simulink model "MCSI_simulation_2024_final_sim"  (R2021a)
settings: Solver=VariableStepAuto  StartTime=0.0  StopTime=10/cfg.fl  RelTol=1e-3
undefined symbols (not defined in the file or in its folder): cfg
libraries: spsIdealSwitchLib x18, simulink x17, hdlsllib x12, spsSeriesRLCBranchLib x8, spsCurrentMeasurementLib x6, commutil2 x6, spsMosfetLib x4, spsTriangleGeneratorLib x3, spsThreePhaseProgrammableGeneratorLib x3, spsMeanLib x2, spsThreePhaseSeriesRLCBranchLib x2, spsThreePhaseVIMeasurementLib x2
(part 2 of 2)

== system MCSI_simulation_2024_final_sim/SPWM_3mod_hdl/tabla_spwm_g1/Decoder ==
  note: LSB
  b2 : Inport
  b1 : Inport  Port=2
  b0 (LSB) : Inport  Port=3
  Logical Operator{,1..7} (8 alike) : Logic  Inputs=3  IconShape=distinctive  AllPortsSameDT=off  OutDataTypeStr=boolean
  Logical Operator10 : Logic  Operator=NOT  IconShape=distinctive  AllPortsSameDT=off  OutDataTypeStr=boolean
  Logical Operator8 : Logic  Operator=NOT  IconShape=distinctive  AllPortsSameDT=off  OutDataTypeStr=boolean
  Logical Operator9 : Logic  Operator=NOT  IconShape=distinctive  AllPortsSameDT=off  OutDataTypeStr=boolean
  Out1 : Outport
  Out2 : Outport  Port=2
  Out3 : Outport  Port=3
  Out4 : Outport  Port=4
  Out5 : Outport  Port=5
  Out6 : Outport  Port=6
  Out7 : Outport  Port=7
  Out8 : Outport  Port=8
  wires:
  Logical Operator9/1 -> Logical Operator5/2, Logical Operator4/2, Logical Operator1/2, Logical Operator/2
  Logical Operator5/1 -> Out6/1
  Logical Operator1/1 -> Out2/1
  Logical Operator10/1 -> Logical Operator3/3, Logical Operator2/3, Logical Operator/3, Logical Operator1/3
  Logical Operator/1 -> Out1/1
  Logical Operator8/1 -> Logical Operator6/1, Logical Operator4/1, Logical Operator2/1, Logical Operator/1
  b2/1 -> Logical Operator4/3, Logical Operator5/3, Logical Operator7/3, Logical Operator6/3, Logical Operator10/1
  b0 (LSB)/1 -> Logical Operator7/1, Logical Operator5/1, Logical Operator3/1, Logical Operator1/1, Logical Operator8/1
  Logical Operator7/1 -> Out8/1
  b1/1 -> Logical Operator3/2, Logical Operator2/2, Logical Operator7/2, Logical Operator6/2, Logical Operator9/1
  Logical Operator4/1 -> Out5/1
  Logical Operator6/1 -> Out7/1
  Logical Operator3/1 -> Out4/1
  Logical Operator2/1 -> Out3/1

== system MCSI_simulation_2024_final_sim/SPWM_3mod_hdl1/Maximum Calculator/Decoder ==
  note: LSB
  b2 : Inport
  b1 : Inport  Port=2
  b0 (LSB) : Inport  Port=3
  Logical Operator{,1..7} (8 alike) : Logic  Inputs=3  IconShape=distinctive  AllPortsSameDT=off  OutDataTypeStr=boolean
  Logical Operator10 : Logic  Operator=NOT  IconShape=distinctive  AllPortsSameDT=off  OutDataTypeStr=boolean
  Logical Operator8 : Logic  Operator=NOT  IconShape=distinctive  AllPortsSameDT=off  OutDataTypeStr=boolean
  Logical Operator9 : Logic  Operator=NOT  IconShape=distinctive  AllPortsSameDT=off  OutDataTypeStr=boolean
  Out1 : Outport
  Out2 : Outport  Port=2
  Out3 : Outport  Port=3
  Out4 : Outport  Port=4
  Out5 : Outport  Port=5
  Out6 : Outport  Port=6
  Out7 : Outport  Port=7
  Out8 : Outport  Port=8
  wires:
  Logical Operator9/1 -> Logical Operator5/2, Logical Operator4/2, Logical Operator1/2, Logical Operator/2
  Logical Operator5/1 -> Out6/1
  Logical Operator1/1 -> Out2/1
  Logical Operator10/1 -> Logical Operator3/3, Logical Operator2/3, Logical Operator/3, Logical Operator1/3
  Logical Operator/1 -> Out1/1
  Logical Operator8/1 -> Logical Operator6/1, Logical Operator4/1, Logical Operator2/1, Logical Operator/1
  b2/1 -> Logical Operator4/3, Logical Operator5/3, Logical Operator7/3, Logical Operator6/3, Logical Operator10/1
  b0 (LSB)/1 -> Logical Operator7/1, Logical Operator5/1, Logical Operator3/1, Logical Operator1/1, Logical Operator8/1
  Logical Operator7/1 -> Out8/1
  b1/1 -> Logical Operator3/2, Logical Operator2/2, Logical Operator7/2, Logical Operator6/2, Logical Operator9/1
  Logical Operator4/1 -> Out5/1
  Logical Operator6/1 -> Out7/1
  Logical Operator3/1 -> Out4/1
  Logical Operator2/1 -> Out3/1

== system MCSI_simulation_2024_final_sim/SPWM_3mod_hdl1/tabla_spwm_g1/Decoder ==
  note: LSB
  b2 : Inport
  b1 : Inport  Port=2
  b0 (LSB) : Inport  Port=3
  Logical Operator{,1..7} (8 alike) : Logic  Inputs=3  IconShape=distinctive  AllPortsSameDT=off  OutDataTypeStr=boolean
  Logical Operator10 : Logic  Operator=NOT  IconShape=distinctive  AllPortsSameDT=off  OutDataTypeStr=boolean
  Logical Operator8 : Logic  Operator=NOT  IconShape=distinctive  AllPortsSameDT=off  OutDataTypeStr=boolean
  Logical Operator9 : Logic  Operator=NOT  IconShape=distinctive  AllPortsSameDT=off  OutDataTypeStr=boolean
  Out1 : Outport
  Out2 : Outport  Port=2
  Out3 : Outport  Port=3
  Out4 : Outport  Port=4
  Out5 : Outport  Port=5
  Out6 : Outport  Port=6
  Out7 : Outport  Port=7
  Out8 : Outport  Port=8
  wires:
  Logical Operator9/1 -> Logical Operator5/2, Logical Operator4/2, Logical Operator1/2, Logical Operator/2
  Logical Operator5/1 -> Out6/1
  Logical Operator1/1 -> Out2/1
  Logical Operator10/1 -> Logical Operator3/3, Logical Operator2/3, Logical Operator/3, Logical Operator1/3
  Logical Operator/1 -> Out1/1
  Logical Operator8/1 -> Logical Operator6/1, Logical Operator4/1, Logical Operator2/1, Logical Operator/1
  b2/1 -> Logical Operator4/3, Logical Operator5/3, Logical Operator7/3, Logical Operator6/3, Logical Operator10/1
  b0 (LSB)/1 -> Logical Operator7/1, Logical Operator5/1, Logical Operator3/1, Logical Operator1/1, Logical Operator8/1
  Logical Operator7/1 -> Out8/1
  b1/1 -> Logical Operator3/2, Logical Operator2/2, Logical Operator7/2, Logical Operator6/2, Logical Operator9/1
  Logical Operator4/1 -> Out5/1
  Logical Operator6/1 -> Out7/1
  Logical Operator3/1 -> Out4/1
  Logical Operator2/1 -> Out3/1

== system MCSI_simulation_2024_final_sim/SPWM_3mod_hdl2/Maximum Calculator/Decoder ==
  note: LSB
  b2 : Inport
  b1 : Inport  Port=2
  b0 (LSB) : Inport  Port=3
  Logical Operator{,1..7} (8 alike) : Logic  Inputs=3  IconShape=distinctive  AllPortsSameDT=off  OutDataTypeStr=boolean
  Logical Operator10 : Logic  Operator=NOT  IconShape=distinctive  AllPortsSameDT=off  OutDataTypeStr=boolean
  Logical Operator8 : Logic  Operator=NOT  IconShape=distinctive  AllPortsSameDT=off  OutDataTypeStr=boolean
  Logical Operator9 : Logic  Operator=NOT  IconShape=distinctive  AllPortsSameDT=off  OutDataTypeStr=boolean
  Out1 : Outport
  Out2 : Outport  Port=2
  Out3 : Outport  Port=3
  Out4 : Outport  Port=4
  Out5 : Outport  Port=5
  Out6 : Outport  Port=6
  Out7 : Outport  Port=7
  Out8 : Outport  Port=8
  wires:
  Logical Operator9/1 -> Logical Operator5/2, Logical Operator4/2, Logical Operator1/2, Logical Operator/2
  Logical Operator5/1 -> Out6/1
  Logical Operator1/1 -> Out2/1
  Logical Operator10/1 -> Logical Operator3/3, Logical Operator2/3, Logical Operator/3, Logical Operator1/3
  Logical Operator/1 -> Out1/1
  Logical Operator8/1 -> Logical Operator6/1, Logical Operator4/1, Logical Operator2/1, Logical Operator/1
  b2/1 -> Logical Operator4/3, Logical Operator5/3, Logical Operator7/3, Logical Operator6/3, Logical Operator10/1
  b0 (LSB)/1 -> Logical Operator7/1, Logical Operator5/1, Logical Operator3/1, Logical Operator1/1, Logical Operator8/1
  Logical Operator7/1 -> Out8/1
  b1/1 -> Logical Operator3/2, Logical Operator2/2, Logical Operator7/2, Logical Operator6/2, Logical Operator9/1
  Logical Operator4/1 -> Out5/1
  Logical Operator6/1 -> Out7/1
  Logical Operator3/1 -> Out4/1
  Logical Operator2/1 -> Out3/1

== system MCSI_simulation_2024_final_sim/SPWM_3mod_hdl2/tabla_spwm_g1/Decoder ==
  note: LSB
  b2 : Inport
  b1 : Inport  Port=2
  b0 (LSB) : Inport  Port=3
  Logical Operator{,1..7} (8 alike) : Logic  Inputs=3  IconShape=distinctive  AllPortsSameDT=off  OutDataTypeStr=boolean
  Logical Operator10 : Logic  Operator=NOT  IconShape=distinctive  AllPortsSameDT=off  OutDataTypeStr=boolean
  Logical Operator8 : Logic  Operator=NOT  IconShape=distinctive  AllPortsSameDT=off  OutDataTypeStr=boolean
  Logical Operator9 : Logic  Operator=NOT  IconShape=distinctive  AllPortsSameDT=off  OutDataTypeStr=boolean
  Out1 : Outport
  Out2 : Outport  Port=2
  Out3 : Outport  Port=3
  Out4 : Outport  Port=4
  Out5 : Outport  Port=5
  Out6 : Outport  Port=6
  Out7 : Outport  Port=7
  Out8 : Outport  Port=8
  wires:
  Logical Operator9/1 -> Logical Operator5/2, Logical Operator4/2, Logical Operator1/2, Logical Operator/2
  Logical Operator5/1 -> Out6/1
  Logical Operator1/1 -> Out2/1
  Logical Operator10/1 -> Logical Operator3/3, Logical Operator2/3, Logical Operator/3, Logical Operator1/3
  Logical Operator/1 -> Out1/1
  Logical Operator8/1 -> Logical Operator6/1, Logical Operator4/1, Logical Operator2/1, Logical Operator/1
  b2/1 -> Logical Operator4/3, Logical Operator5/3, Logical Operator7/3, Logical Operator6/3, Logical Operator10/1
  b0 (LSB)/1 -> Logical Operator7/1, Logical Operator5/1, Logical Operator3/1, Logical Operator1/1, Logical Operator8/1
  Logical Operator7/1 -> Out8/1
  b1/1 -> Logical Operator3/2, Logical Operator2/2, Logical Operator7/2, Logical Operator6/2, Logical Operator9/1
  Logical Operator4/1 -> Out5/1
  Logical Operator6/1 -> Out7/1
  Logical Operator3/1 -> Out4/1
  Logical Operator2/1 -> Out3/1
